simulink model "shuzijidai2fsk"  (Simulink 6.0)
settings: Solver=ode45  StartTime=0.0  StopTime=5  RelTol=1e-3
libraries: dsparch4 x4, commchan2 x1, commrandsrc2 x1
settings Model: LastModifiedBy=xxgcxy602

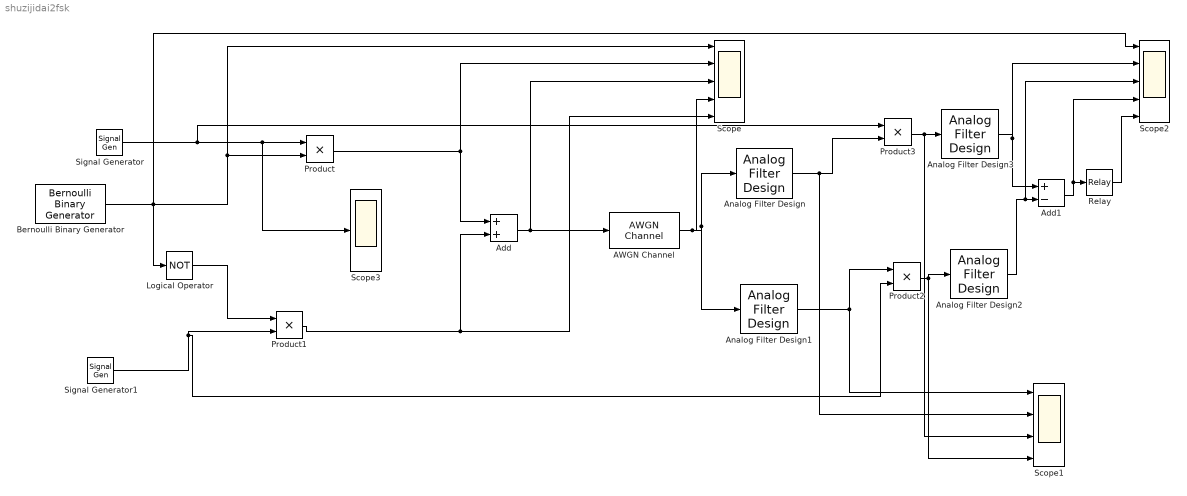
== system shuzijidai2fsk ==
  AWGN Channel : commchan2/AWGN Channel  seed=67  noiseMode=Variance from mask  EbNodB=10  EsNodB=10  SNRdB=10  bitsPerSym=1  Ps=1  Tsym=1  variance=1
  Add : Sum  OutScaling=2^-10
  Add1 : Sum  Inputs=+-  OutScaling=2^-10
  Analog Filter Design : dsparch4/Analog Filter Design  method=Butterworth  filttype=Bandpass  N=8  Wlo=2*pi*280  Whi=2*pi*320  Rp=2  Rs=40
  Analog Filter Design1 : dsparch4/Analog Filter Design  method=Butterworth  filttype=Bandpass  N=8  Wlo=2*pi*80  Whi=2*pi*120  Rp=2  Rs=40
  Analog Filter Design2 : dsparch4/Analog Filter Design  method=Butterworth  filttype=Lowpass  N=2  Wlo=2*pi*7  Whi=80  Rp=2  Rs=40
  Analog Filter Design3 : dsparch4/Analog Filter Design  method=Butterworth  filttype=Lowpass  N=2  Wlo=2*pi*7  Whi=80  Rp=2  Rs=40
  Bernoulli Binary Generator : commrandsrc2/Bernoulli Binary Generator  P=0.5  seed=61  Ts=0.5  frameBased=off  sampPerFrame=1  orient=off
  Logical Operator : Logic  Operator=NOT  AllPortsSameDT=off  OutDataTypeMode=Boolean
  Product{,1..3} (4 alike) : Product  RndMeth=Zero
  Relay : Relay  OnSwitchValue=0.5  OffSwitchValue=0.5
  Scope : Scope  NumInputPorts=5
      settings: YMin=-5~-5~-5~-5~-5  YMax=5~5~5~5~5
  Scope1 : Scope  NumInputPorts=4
      settings: YMin=-5~-5~-5~-5  YMax=5~5~5~5
  Scope2 : Scope  NumInputPorts=5
      settings: YMin=-5~-5~-5~-5~-5  YMax=5~5~5~5~5  SaveName=ScopeData2
  Scope3 : Scope
      settings: SaveName=ScopeData3
  Signal Generator : SignalGenerator  Amplitude=2  Frequency=2*pi*300  Units=rad/sec
  Signal Generator1 : SignalGenerator  Amplitude=2  Frequency=2*pi*100  Units=rad/sec
  wires:
  Signal Generator/1 -> Product3/1, Product/1, Scope3/1
  Product1/1 -> Scope/5, Add/2
  Bernoulli Binary Generator/1 -> Scope/1, Product/2, Logical Operator/1, Scope2/1
  Product/1 -> Add/1, Scope/2
  AWGN Channel/1 -> Analog Filter Design/1, Analog Filter Design1/1, Scope/4
  Analog Filter Design1/1 -> Product2/1, Scope1/1
  Logical Operator/1 -> Product1/1
  Signal Generator1/1 -> Product1/2, Product2/2
  Analog Filter Design/1 -> Product3/2, Scope1/2
  Product2/1 -> Analog Filter Design2/1, Scope1/4
  Product3/1 -> Analog Filter Design3/1, Scope1/3
  Analog Filter Design3/1 -> Add1/1, Scope2/2
  Analog Filter Design2/1 -> Add1/2, Scope2/3
  Add1/1 -> Relay/1, Scope2/4
  Relay/1 -> Scope2/5
  Add/1 -> AWGN Channel/1, Scope/3
